simulink model "VCU_F407"  (R2026a)
settings: Solver=FixedStepDiscrete  StopTime=inf  FixedStep=0.001  EnableMultiTasking=on
libraries: stm32blockslib x1
settings Model: STM32="{\"DigitalPortWrite\":{\"ID\":\"11\"}}"  Creator=1011472417  LastModifiedBy=1011472417
settings SolverCC: PositivePriorityOrder=on
settings HardwareCC: ProdLargestAtomicInteger=Long  ProdLargestAtomicFloat=Double  ProdHWDeviceType=ARM Compatible->ARM Cortex-M
settings RTWCC: SystemTargetFile=ert.tlc  HardwareBoard=STM32F4xx Based  TLCOptions=-aInlineSetEventsForThisBaseRateFcn=TLC_FALSE -aSuppressMultiTaskScheduler=TLC_FALSE -aRateBasedStepFcn=1  Toolchain=GNU Tools for STM32  BuildConfiguration=Faster Runs  Description=Embedded Coder
settings ERTTargetCC: ExtModeTransport=3.0  ExtModeStaticAllocSize=2048.0  CodeReplacementLibrary=ARM Cortex-M

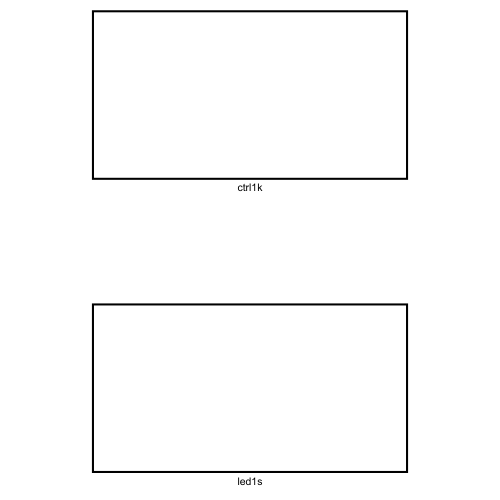
[thumbnail: Simulink's stored preview of the top-level diagram]
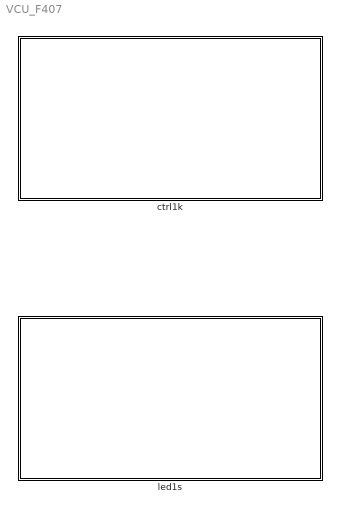
== system VCU_F407 ==
  ctrl1k : Subsystem  TreatAsAtomicUnit=on  SystemSampleTime=0.001
  led1s : Subsystem  TreatAsAtomicUnit=on  SystemSampleTime=1.0

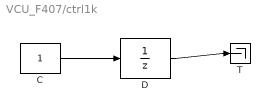
== system VCU_F407/ctrl1k ==
  C : Constant
  D : UnitDelay  SampleTime=0.001
  T : Terminator
  wires:
  C/1 -> D/1
  D/1 -> T/1

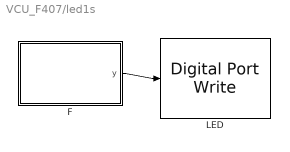
== system VCU_F407/led1s ==
  F : MATLAB Function  TreatAsAtomicUnit=on
  LED : stm32blockslib/Digital Port Write  PortName=GPIOD  PinNumber=[0 1]  ReadOperation=off  IOAsArray=on  SampleTime=-1
  wires:
  F/1(y) -> LED/1

== matlab function VCU_F407/led1s/F ==
  data: y output
function y = led_toggle()
%#codegen
persistent s
if isempty(s)
    s = false;
end
s = ~s;
y = [s; s];
end
